simulink model "demo_rt"  (R2020b)
settings: Solver=VariableStepAuto  StartTime=0.0  StopTime=10.0  RelTol=1e-3
settings Model: Creator=ThinkPad  LastModifiedBy=ThinkPad

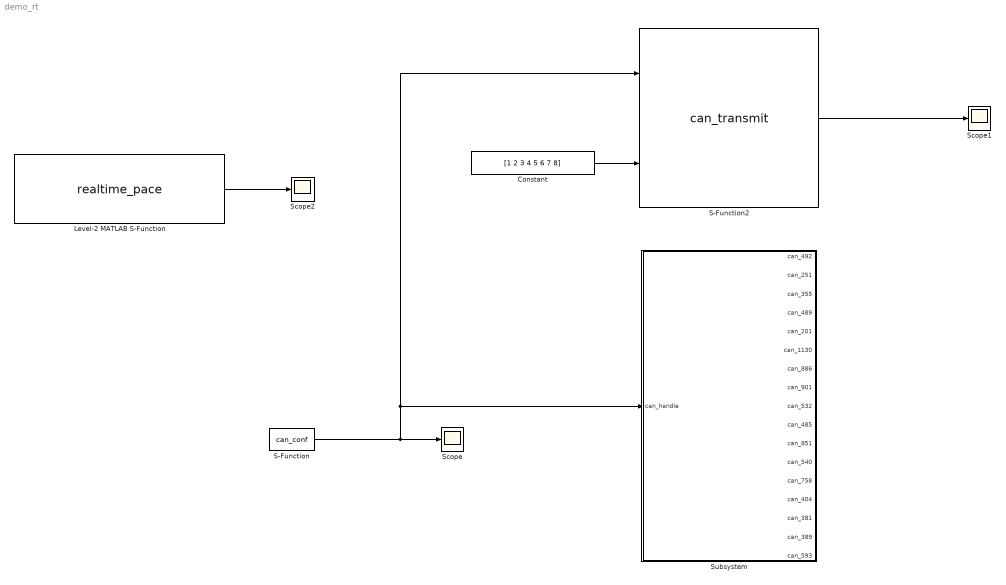
== system demo_rt ==
  Constant : Constant  Value=[1 2 3 4 5 6 7 8]  OutDataTypeStr=uint8
  Level-2 MATLAB S-Function : M-S-Function  FunctionName=realtime_pace  Parameters=1
  S-Function : S-Function  FunctionName=can_conf  SFunctionDeploymentMode=off  EnableBusSupport=off
  S-Function2 : S-Function  FunctionName=can_transmit  Parameters=509  SFunctionDeploymentMode=off  EnableBusSupport=off
  Scope : Scope
  Scope1 : Scope
  Scope2 : Scope
  Subsystem : Subsystem
      mask Display: disp('can_read_ZS11');
  wires:
  S-Function/1 -> Subsystem/1(can_handle), S-Function2/1, Scope/1
  Constant/1 -> S-Function2/2
  S-Function2/1 -> Scope1/1
  Level-2 MATLAB S-Function/1 -> Scope2/1

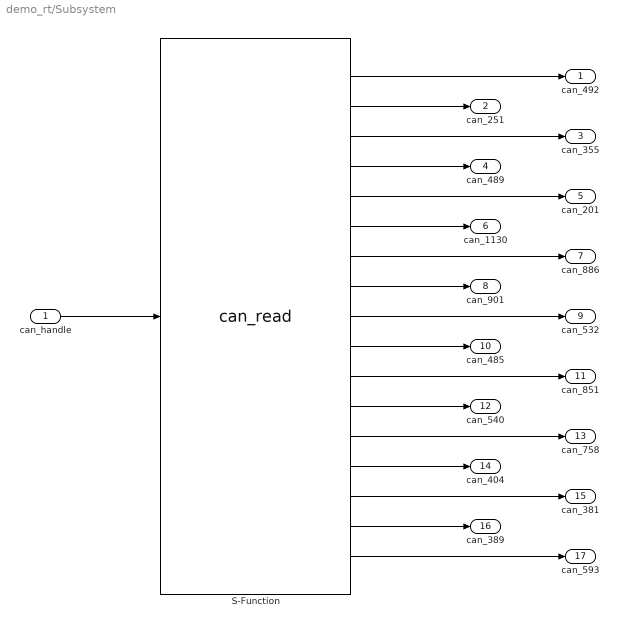
== system demo_rt/Subsystem ==
  can_handle : Inport
  S-Function : S-Function  FunctionName=can_read  SFunctionDeploymentMode=off  EnableBusSupport=off
  can_492 : Outport
  can_251 : Outport  Port=2
  can_355 : Outport  Port=3
  can_489 : Outport  Port=4
  can_201 : Outport  Port=5
  can_1130 : Outport  Port=6
  can_886 : Outport  Port=7
  can_901 : Outport  Port=8
  can_532 : Outport  Port=9
  can_485 : Outport  Port=10
  can_851 : Outport  Port=11
  can_540 : Outport  Port=12
  can_758 : Outport  Port=13
  can_404 : Outport  Port=14
  can_381 : Outport  Port=15
  can_389 : Outport  Port=16
  can_593 : Outport  Port=17
  wires:
  can_handle/1 -> S-Function/1
  S-Function/1 -> can_492/1
  S-Function/2 -> can_251/1
  S-Function/3 -> can_355/1
  S-Function/4 -> can_489/1
  S-Function/5 -> can_201/1
  S-Function/6 -> can_1130/1
  S-Function/7 -> can_886/1
  S-Function/8 -> can_901/1
  S-Function/9 -> can_532/1
  S-Function/10 -> can_485/1
  S-Function/11 -> can_851/1
  S-Function/12 -> can_540/1
  S-Function/13 -> can_758/1
  S-Function/14 -> can_404/1
  S-Function/15 -> can_381/1
  S-Function/16 -> can_389/1
  S-Function/17 -> can_593/1
